simulink subsystem "Coordinator"  (R2023a)
settings: Solver=VariableStepAuto  StartTime=0.0  StopTime=10.0  RelTol=1e-3
settings Model: Creator=Franz  LastModifiedBy=Franz

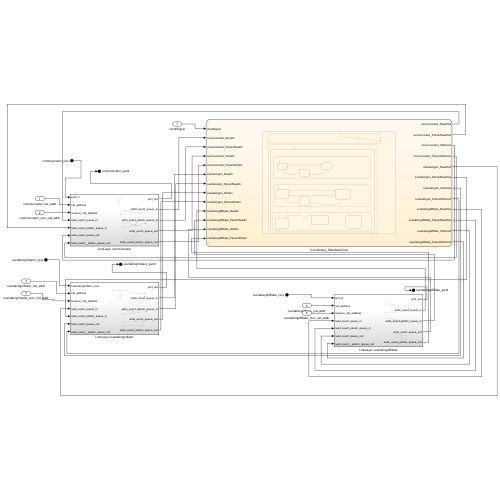
[thumbnail: Simulink's stored preview of the top-level diagram]
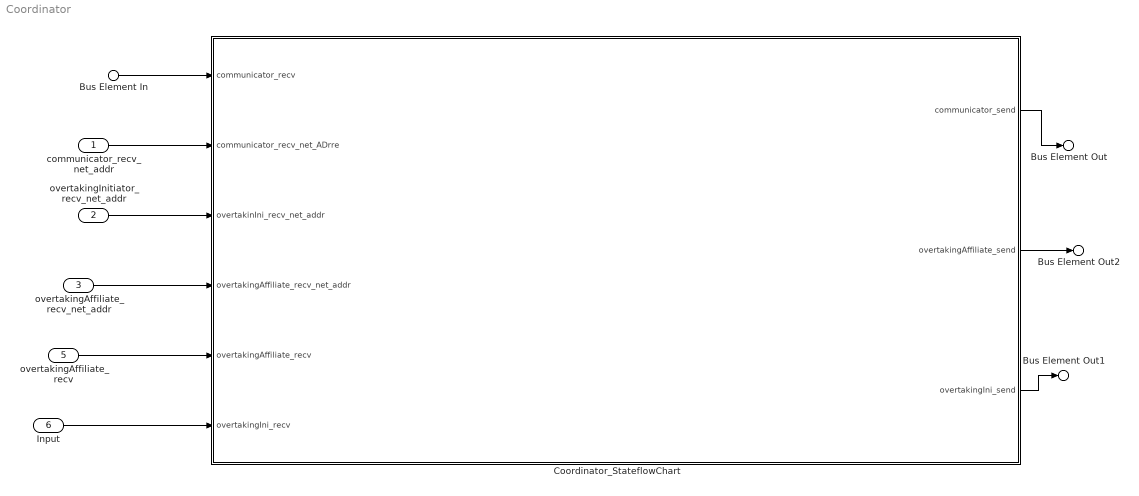
== system Coordinator ==
  communicator_recv_net_addr : Inport
  overtakingInitiator_recv_net_addr : Inport  Port=2
  overtakingAffiliate_recv_net_addr : Inport  Port=3
  Bus Element In : Inport  Port=4  PortName=communicator_recv
  overtakingAffiliate_recv : Inport  Port=5
  Input : Inport  Port=6
  Coordinator_StateflowChart : Stateflow chart  TreatAsAtomicUnit=on
      settings: PortSchema="{\"entries\":[{\"content\":{\"sides\":[{\"content\":{\"connectorIds\":[\"In1\",\"In2\",\"In4\",\"In5\",\"In6\",\"In3\"]},\"type\":\"ConnectorPlacement.EquallySpacedRectSide\",\"uuid\":\"22fb6c1c-8c2a-47a2-a6db-e7859c525a92\"},{\"content\":{\"connectorIds\":[\"Out1\",\"Out2\",\"Out3\"],\"side\":\"RIGHT\"},\"type\":\"ConnectorPlacement.EquallySpacedRectSide\",\"uuid\":\"c43310d7-877a-40f2-b2b4-0121302933cb\"},{\"content\":{\"side\":\"TOP\"},\"type\":\"ConnectorPlacement.EquallySpacedRectSide\",\"uuid\":\"c8b3dcc0-f0ac-4f18-9760-66b96ce6764e\"}]},\"type\":\"ConnectorPlacement.EquallySpacedConnector\",\"uuid\":\"ff2397da-a624-4aae-9f08-1bcd4ebe3cb3\"}],\"packageUris\":[\"http://schema.mathworks.com/mf0/Connector/R2020b\"],\"version\":\"1.0\"}"
  Bus Element Out : Outport  PortName=communicator_send
  Bus Element Out1 : Outport  Port=2  PortName=overtakingInitiator_send
  Bus Element Out2 : Outport  Port=3  PortName=overtakingAffiliate_send
  wires:
  communicator_recv_net_addr/1 -> Coordinator_StateflowChart/2(communicator_recv_net_ADrre)
  overtakingAffiliate_recv_net_addr/1 -> Coordinator_StateflowChart/5(overtakingAffiliate_recv_net_addr)
  Bus Element In/1 -> Coordinator_StateflowChart/1(communicator_recv)
  Coordinator_StateflowChart/1(communicator_send) -> Bus Element Out/1
  overtakingInitiator_recv_net_addr/1 -> Coordinator_StateflowChart/4(overtakinIni_recv_net_addr)
  Coordinator_StateflowChart/2(overtakingAffiliate_send) -> Bus Element Out2/1
  Coordinator_StateflowChart/3(overtakingIni_send) -> Bus Element Out1/1
  overtakingAffiliate_recv/1 -> Coordinator_StateflowChart/6(overtakingAffiliate_recv)
  Input/1 -> Coordinator_StateflowChart/3(overtakingIni_recv)

== stateflow chart Coordinator/Coordinator_StateflowChart ==
  state chart
    state chartRegion [parallel]
      settings: executionOrder=1
      state Coordinator_main
        state communicatorPort [parallel]
          settings: executionOrder=3
          state Idle
          state WaitForCoordinator
          state WaitForOvertaking
          (default) -> chart.chartRegion.Coordinator_main.communicatorPort.Idle
          chart.chartRegion.Coordinator_main.communicatorPort.Idle -> WaitForCoordinator : [communicator_recv==1 && coordination_Succesfull == false]{send(overtakingRequested, overtakingInitPort); coordination_Succesfull =true}
          WaitForCoordinator -> chart.chartRegion.Coordinator_main.communicatorPort.Idle [order 2] : denyPermission{communicator_send=4}
          WaitForCoordinator -> WaitForOvertaking [order 1] : grantPermission{communicator_send=1}
          WaitForOvertaking -> chart.chartRegion.Coordinator_main.communicatorPort.Idle : [communicator_recv == 2]{send(executedOvertaking,overtakingInitPort)}
        state overtakingInitPort [parallel]
          settings: executionOrder=2
          state Initiating
          state Idle
          state Passing
          chart.chartRegion.Coordinator_main.overtakingInitPort.Idle -> Initiating : overtakingRequested[boolean_coordinationbusy == false]{overtakingIni_send=1}
          (default) -> chart.chartRegion.Coordinator_main.overtakingInitPort.Idle
          Initiating -> chart.chartRegion.Coordinator_main.overtakingInitPort.Idle [order 1] : requestOvertaking
          Initiating -> Passing [order 2] : [overtakingIni_recv == 1]{send(grantPermission, communicatorPort )}
          Passing -> chart.chartRegion.Coordinator_main.overtakingInitPort.Idle : executedOvertaking{overtakingIni_send= 2 }
        state overtakingAffiliatePort [parallel]
          settings: executionOrder=1
          state Coordinating
          state GettingPassed
          state Idle
          chart.chartRegion.Coordinator_main.overtakingAffiliatePort.Idle -> Coordinating : [overtakingAffiliate_recv == 1 && boolean_coordinationbusy == false ]{boolean_coordinationbusy=true; }
          (default) -> chart.chartRegion.Coordinator_main.overtakingAffiliatePort.Idle
          Coordinating -> GettingPassed : {overtakingAffiliate_send=1}
          GettingPassed -> chart.chartRegion.Coordinator_main.overtakingAffiliatePort.Idle : [overtakingAffiliate_recv == 2]{boolean_coordinationbusy = false}
      (default) -> Coordinator_main
  note: OvertakingRequested: communicator_recv == 1
      | overtakingSuccessfull: communicator_recv == 2
      |
      |
      | grantPermission: communicator_send = 1
      | denyPermission: communicator_send = 4
      |
      |
      | overtakingRequested: overtakingIni_send = 1
      | executedOvertaking: overtakingIni_send = 2
      |
      |
      | acceptedOvertaking: overtakingIni_recv == 1
      |
      |
      | overtakingRequested: overtakingAffiliate_recv == 1
      | overtakingFinished: overtakingAffiliate_rev == 2
  (default) -> chart
  data: communicator_recv input; communicator_recv_net_ADrre input; int32_coordinationTimeout local int32; boolean_coordinationbusy local boolean =false; communicator_send output double; overtakingIni_recv input int32; overtakinIni_recv_net_addr input; overtakingAffiliate_recv_net_addr input; overtakingAffiliate_recv input; overtakingAffiliate_send output int32; overtakingIni_send output int32; coordination_Succesfull local =false
  events: requestPermission local FUNCTION_CALL_EVENT; overtakingRequested local FUNCTION_CALL_EVENT; denyPermission local FUNCTION_CALL_EVENT; grantPermission local FUNCTION_CALL_EVENT; coordinationSuccessful local FUNCTION_CALL_EVENT; executedOvertaking local FUNCTION_CALL_EVENT; overtakingSuccessful local FUNCTION_CALL_EVENT; requestOvertaking local FUNCTION_CALL_EVENT; acceptedOvertaling local FUNCTION_CALL_EVENT; finishedOvertaking local FUNCTION_CALL_EVENT; acceptedOvertaking local FUNCTION_CALL_EVENT
